simulink model "Copy_of_Mando"  (R2017b)
settings: Solver=FixedStepDiscrete  StartTime=0.0  StopTime=inf  FixedStep=0.001  MaxStep=1e-4  RelTol=1e-3  EnableMultiTasking=on
undefined symbols (not defined in the file): c_a, c_v, delta, Fc_mas_id, Fc_menos_id, Fs_mas_id, Fs_menos_id, Kp_c1, Kp_c2, Kp_h1, Kp_h2, Kv_c1, Kv_c2, Kv_h1, Kv_h2, nL, precision, sigma0_id, sigma1_id, sigma2_id, tau1, tfin, tini, vs_id
libraries: simulink x9, slrtlib x4, xpcnilib x3, dspbuff3 x2, vrlib x1, powerlib x1
settings Model: Creator=salas  LastModifiedBy=TrendingPC
settings OptimizationCC: LifeSpan=inf
settings DebuggingCC: SFUnexpectedBacktrackingDiag=warning  SFNoUnconditionalDefaultTransitionDiag=warning  SFExecutionAtInitializationDiag=none
settings CodeAppCC: StateflowObjectComments=on
settings GRTTargetCC: TargetLangStandard=C89/C90 (ANSI)  GeneratePreprocessorConditionals=Disable all
settings ConfigComp: CovMetricSettings=dw  CovHtmlReporting=on  CovSaveCumulativeToWorkspaceVar=on  CovSaveSingleToWorkspaceVar=on  CovExternalEMLEnable=off
settings SimscapeCC: SimscapeNormalizeSystem=off

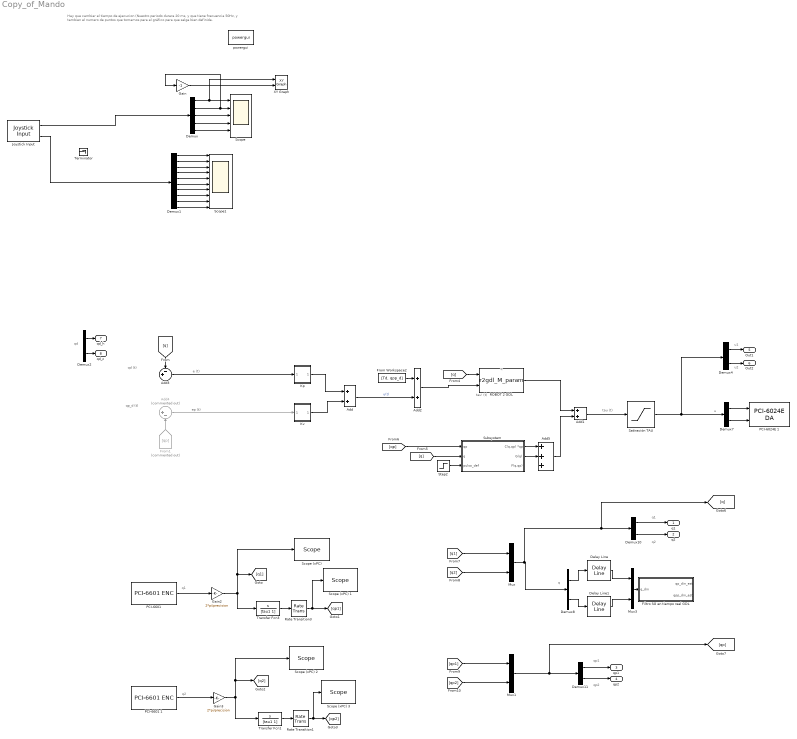
== system Copy_of_Mando ==
  note: Hay que cambiar el tiempo de ejecucion (Nuestro periodo durara 20 ms, y que tiene frecuencia 50Hz, y tambien el numero de puntos que tomamos para el gráfico para que salga bien definida.
  note: qd (t)
  note: q
  note: qd
  note: u1
  note: q2
  note: q2
  note: u2
  note: u
  note: qp2
  note: q1
  note: q
  note: qp_d (t)
  note: tau' (t)
  note: tau (t)
  note: e (t)
  note: q1
  note: ep (t)
  note: qp1
  Add : Sum
  Add1 : Sum
  Add2 : Sum
  Add3 : Sum  Inputs=-+|
  Add4 : Sum  Commented=on  Inputs=|+-
  Add5 : Sum  Inputs=+++
  Delay Line : dspbuff3/Delay Line  siz=nL+1  ic=0  directfeed=on  enable_output=off  hold_output=off  OutputFrames=on
      settings: SourceProductName=DSP System Toolbox  SourceProductBaseCode=DS
  Delay Line1 : dspbuff3/Delay Line  siz=nL+1  ic=0  directfeed=on  enable_output=off  hold_output=off  OutputFrames=on
      settings: SourceProductName=DSP System Toolbox  SourceProductBaseCode=DS
  Demux : Demux  Outputs=5
  Demux1 : Demux  Outputs=10
  Demux{2,4,7..8,10..11} (6 alike) : Demux  Outputs=2
  Filtro SG en tiempo real GDL : Subsystem
  From Workspace2 : FromWorkspace  VariableName=[Td, qpp_d]  SampleTime=0
  From1 : From  Commented=on  GotoTag=qp
      settings: CloseFcn=tagdialog Close
  Gain : Gain  Gain=-1
  Gain2 : Gain  Gain=2*pi/precision
  Gain3 : Gain  Gain=2*pi/precision
  Joystick Input : vrlib/Joystick Input  joyid=1  adjustports=on  forcefeed=off
      settings: SourceProductBaseCode=VR
  Kp : Subsystem
  Kv : Subsystem
  Mux : Mux  Inputs=2
  Mux1 : Mux  Inputs=2
  Mux3 : Mux  Inputs=2
  PCI-6024E 1 : xpcnilib/D//A/E Series/PCI-6024E DA  channel=[1,2]  reset=[1]  initValue=[0]  sampletime=0.001  slot=-1
      settings: SourceProductName=Simulink Real-Time  SourceProductBaseCode=XP
  "PCI-6601 " : xpcnilib/Incremental Encoder/PCI-6601 ENC  channel=1  countMode=Quadrature Mode X1  initCount=0  reload=off  indexPhase=A high B high  filter=None  sampleTime=0.001  slot=-1
      settings: SourceProductName=Simulink Real-Time  SourceProductBaseCode=XP
  PCI-6601 1 : xpcnilib/Incremental Encoder/PCI-6601 ENC  channel=2  countMode=Quadrature Mode X1  initCount=0  reload=off  indexPhase=A high B high  filter=None  sampleTime=0.001  slot=-1
      settings: SourceProductName=Simulink Real-Time  SourceProductBaseCode=XP
  ROBOT 2 GDL : S-Function  FunctionName=r2gdl_M_param  Parameters=k_id  SFunctionDeploymentMode=off  EnableBusSupport=off
  Rate Transition1 : RateTransition  OutPortSampleTime=0.001
  Rate Transition3 : RateTransition  OutPortSampleTime=0.001
  Satiración TAU : Saturate  UpperLimit=10  LowerLimit=-10  SampleTime=0.001
  Scope : Scope  NumInputPorts=5
  "Scope (xPC) " : slrtlib/Displays and Logging/Scope   scopeno=1  scopetype=Target  autostart=on  viewmode=Graphical redraw  formatstr='%15.6f'  grid=on  ylimits=[0,0]  nosamples=250  noprepostsamples=0  interleave=1  triggermode=FreeRun  triggersignal=1  trigsignalfromport=off  triggerlevel=0.0  triggerslope=Either  triggerscope=1  triggersample=0  filename=data.dat  mode=Lazy  writesize=512  autorestart=off  dynamicfilemode=off  maxwritefilesize=512*1024^2
  Scope (xPC) 1 : slrtlib/Displays and Logging/Scope   scopeno=2  scopetype=Target  autostart=on  viewmode=Graphical redraw  formatstr='%15.6f'  grid=on  ylimits=[0,0]  nosamples=250  noprepostsamples=0  interleave=1  triggermode=FreeRun  triggersignal=1  trigsignalfromport=off  triggerlevel=0.0  triggerslope=Either  triggerscope=1  triggersample=0  filename=data.dat  mode=Lazy  writesize=512  autorestart=off  dynamicfilemode=off  maxwritefilesize=512*1024^2
  Scope (xPC) 2 : slrtlib/Displays and Logging/Scope   scopeno=3  scopetype=Target  autostart=on  viewmode=Graphical redraw  formatstr='%15.6f'  grid=on  ylimits=[0,0]  nosamples=250  noprepostsamples=0  interleave=1  triggermode=FreeRun  triggersignal=1  trigsignalfromport=off  triggerlevel=0.0  triggerslope=Either  triggerscope=1  triggersample=0  filename=data.dat  mode=Lazy  writesize=512  autorestart=off  dynamicfilemode=off  maxwritefilesize=512*1024^2
  Scope (xPC) 3 : slrtlib/Displays and Logging/Scope   scopeno=4  scopetype=Target  autostart=on  viewmode=Graphical redraw  formatstr='%15.6f'  grid=on  ylimits=[0,0]  nosamples=250  noprepostsamples=0  interleave=1  triggermode=FreeRun  triggersignal=1  trigsignalfromport=off  triggerlevel=0.0  triggerslope=Either  triggerscope=1  triggersample=0  filename=data.dat  mode=Lazy  writesize=512  autorestart=off  dynamicfilemode=off  maxwritefilesize=512*1024^2
  Scope1 : Scope  NumInputPorts=10
  Step2 : Step  Time=0  SampleTime=0.001
  Subsystem : Subsystem
  Terminator : Terminator
  Transfer Fcn1 : TransferFcn  Numerator=[1 0]  Denominator=[tau1 1]
  Transfer Fcn3 : TransferFcn  Numerator=[1 0]  Denominator=[tau1 1]
  XY Graph : simulink/Sinks/XY Graph  xmin=-1  xmax=1  ymin=-1  ymax=1  st=-1
  powergui : powerlib/powergui  Priority=1  SimulationMode=Discrete  SampleTime=0.001  frequency=60  Iterations=50  frequencyindice=50  Pbase=100e6  ErrMax=1e-4  UnitsV=kV  UnitsW=MW  buscounter=0  FunctionMessages=off  echomessages=off  EnableUseOfTLC=off  CurrentSourceSwitches=off  DisableSnubberDevices=off  DisableRonSwitches=off  DisableVfSwitches=off  DisplayEquations=off  SolverType=Tustin/Backward Euler (TBE)  Interpol=off  ExternalGateDelay=off  methode=off  Ts=100  x0status=blocks  SPID=on  SwTol=0  HookPort=off  RestoreLinks=warning  ResistiveCurrentMeasurement=off  Frange=[0:2:500]  Ylog=off  Xlog=on  ShowGrid=off  save=off  variable=ZData  structure=0  ZoomFFT=off  StartTime=0.0  cycles=1  DisplayStyle=1  fundamental=60  FreqAxis=off  MaxFrequency=1000  frequencyindicesteady=1  RmsSteady=1  display=off
  q1 : Outport
  q2 : Outport  Port=2
  qp1 : Outport  Port=3
  qp2 : Outport  Port=4
  Out1 : Outport  Port=5
  Out2 : Outport  Port=6
  qd_h : Outport  Port=7
  qd_c : Outport  Port=8
  wires:
  Joystick Input/1 -> Demux/1
  Demux/1 -> XY Graph/1, Scope/1
  Demux/3 -> Scope/3
  Demux/4 -> Scope/4
  Demux/5 -> Scope/5
  Gain/1 -> XY Graph/2
  Demux/2 -> Gain/1, Scope/2
  Demux1/1 -> Scope1/1
  Demux1/2 -> Scope1/2
  Demux1/3 -> Scope1/3
  Demux1/4 -> Scope1/4
  Demux1/5 -> Scope1/5
  Demux1/6 -> Scope1/6
  Demux1/7 -> Scope1/7
  Demux1/8 -> Scope1/8
  Demux1/9 -> Scope1/9
  Demux1/10 -> Scope1/10
  Joystick Input/2 -> Demux1/1
  ? -> Terminator/1
  Demux10/1 -> q1/1
  Demux11/2 -> qp2/1
  Kv/1(Kp*e) -> Add/2
  "PCI-6601 "/1 -> Gain2/1
  Demux8/2 -> Delay Line1/1
  Demux7/1 -> PCI-6024E 1/1
  Rate Transition3/1 -> Scope (xPC) 1/1, [qp1]
  Mux1/1 -> [qp], Demux11/1
  Mux3/1 -> Filtro SG en tiempo real GDL/1(q_din)
  Add5/1 -> Add1/2
  Demux10/2 -> q2/1
  Transfer Fcn1/1 -> Rate Transition1/1
  [q] -> Add3/1
  [qp1] -> Mux1/1
  ? -> Demux2/1, Add3/2
  Gain2/1 -> Transfer Fcn3/1, "Scope (xPC) "/1, [q1]
  Demux2/1 -> qd_h/1
  [q] -> ROBOT 2 GDL/1
  Mux/1 -> Demux10/1, [q], Demux8/1
  Demux4/1 -> Out1/1
  Rate Transition1/1 -> Scope (xPC) 3/1, [qp2]
  Transfer Fcn3/1 -> Rate Transition3/1
  Delay Line/1 -> Mux3/1
  [qp2] -> Mux1/2
  Delay Line1/1 -> Mux3/2
  PCI-6601 1/1 -> Gain3/1
  [q2] -> Mux/2
  Demux8/1 -> Delay Line/1
  Demux2/2 -> qd_c/1
  Gain3/1 -> [q2], Scope (xPC) 2/1, Transfer Fcn1/1
  Subsystem/1(C(q,qp) *qp) -> Add5/1
  ROBOT 2 GDL/1 -> Add1/1
  Satiración TAU/1 -> Demux4/1, Demux7/1
  ? -> Add4/1
  Add2/1 -> ROBOT 2 GDL/2
  Demux7/2 -> PCI-6024E 1/2
  [qp] -> Subsystem/1(qp)
  Add3/1 -> Kp/1(e(t))
  Step2/1 -> Subsystem/3(pulso_def)
  Add/1 -> Add2/2  "u(t)"
  Demux4/2 -> Out2/1
  Add1/1 -> Satiración TAU/1
  Add4/1 -> Kv/1(e(t))
  Kp/1(Kp*e) -> Add/1
  [q1] -> Mux/1
  [q] -> Subsystem/2(q)
  Demux11/1 -> qp1/1
  From Workspace2/1 -> Add2/1
  Subsystem/2(G(q)) -> Add5/2
  From1/1 -> Add4/2

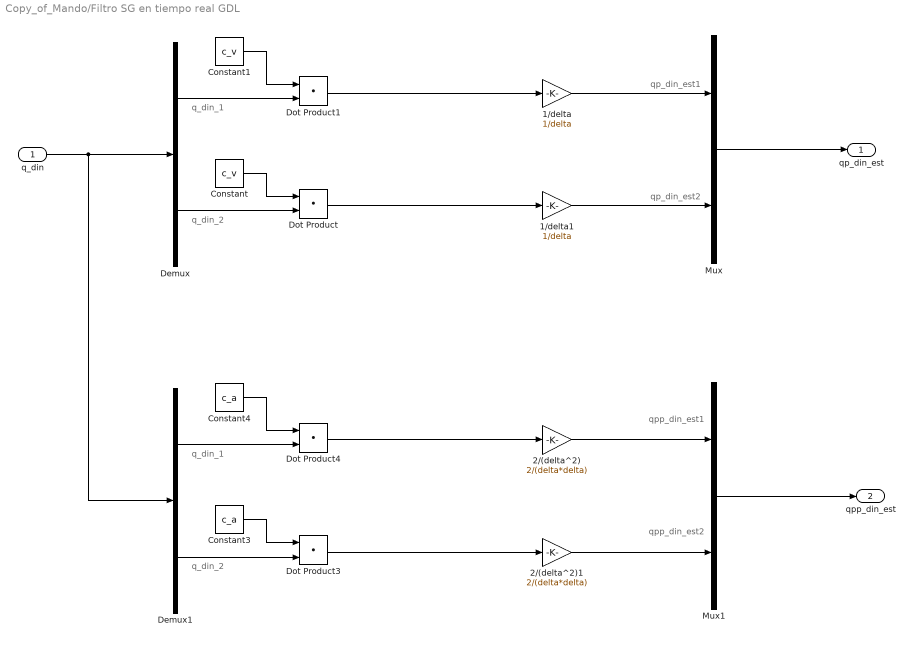
== system Copy_of_Mando/Filtro SG en tiempo real GDL ==
  note: q_din_2
  note: q_din_1
  note: qp_din_est1
  note: qp_din_est2
  note: q_din_2
  note: q_din_1
  note: qpp_din_est1
  note: qpp_din_est2
  q_din : Inport  SampleTime=0.001
  1/delta : Gain  Gain=1/delta  SampleTime=0.001
  1/delta1 : Gain  Gain=1/delta  SampleTime=0.001
  2/(delta^2) : Gain  Gain=2/(delta*delta)  SampleTime=0.001
  2/(delta^2)1 : Gain  Gain=2/(delta*delta)  SampleTime=0.001
  Constant : Constant  Value=c_v  SampleTime=0.001
  Constant1 : Constant  Value=c_v  SampleTime=0.001
  Constant3 : Constant  Value=c_a  VectorParams1D=off  SampleTime=0.001
  Constant4 : Constant  Value=c_a  SampleTime=0.001
  Demux : Demux  Outputs=2
  Demux1 : Demux  Outputs=2
  Dot Product{,1,3..4} (4 alike) : DotProduct  InputSameDT=on  OutDataTypeStr=Inherit: Inherit via internal rule
  Mux : Mux  Inputs=2
  Mux1 : Mux  Inputs=2
  qp_din_est : Outport  SampleTime=0.001
  qpp_din_est : Outport  Port=2  SampleTime=0.001
  wires:
  q_din/1 -> Demux/1, Demux1/1
  Constant1/1 -> Dot Product1/1
  Demux/1 -> Dot Product1/2
  1/delta/1 -> Mux/1
  1/delta1/1 -> Mux/2
  Mux/1 -> qp_din_est/1
  Dot Product/1 -> 1/delta1/1
  Dot Product1/1 -> 1/delta/1
  Demux/2 -> Dot Product/2
  Constant/1 -> Dot Product/1
  Constant4/1 -> Dot Product4/1
  Demux1/1 -> Dot Product4/2
  2/(delta^2)/1 -> Mux1/1
  2/(delta^2)1/1 -> Mux1/2
  Dot Product3/1 -> 2/(delta^2)1/1
  Dot Product4/1 -> 2/(delta^2)/1
  Demux1/2 -> Dot Product3/2
  Constant3/1 -> Dot Product3/1
  Mux1/1 -> qpp_din_est/1

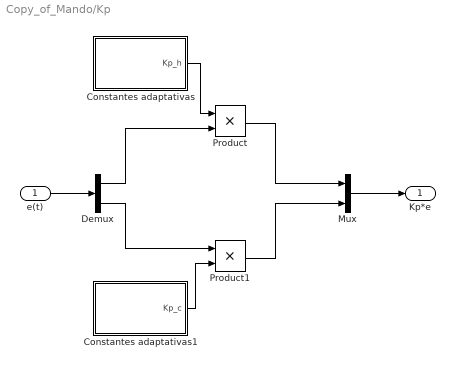
== system Copy_of_Mando/Kp ==
  e(t) : Inport
  Constantes adaptativas : Subsystem
  Constantes adaptativas1 : Subsystem
  Demux : Demux  Outputs=2
  Mux : Mux  Inputs=2
  Product : Product  RndMeth=Zero
  Product1 : Product  RndMeth=Zero
  Kp*e : Outport
  wires:
  Constantes adaptativas1/1(Kp_c) -> Product1/2
  Demux/2 -> Product1/1
  Product1/1 -> Mux/2
  Constantes adaptativas/1(Kp_h) -> Product/1
  Product/1 -> Mux/1
  Demux/1 -> Product/2
  Mux/1 -> Kp*e/1
  e(t)/1 -> Demux/1

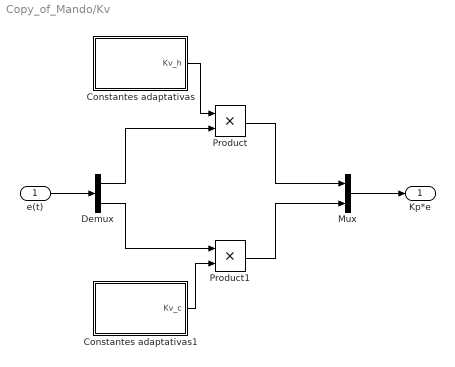
== system Copy_of_Mando/Kv ==
  e(t) : Inport
  Constantes adaptativas : Subsystem
  Constantes adaptativas1 : Subsystem
  Demux : Demux  Outputs=2
  Mux : Mux  Inputs=2
  Product : Product  RndMeth=Zero
  Product1 : Product  RndMeth=Zero
  Kp*e : Outport
  wires:
  e(t)/1 -> Demux/1
  Mux/1 -> Kp*e/1
  Demux/1 -> Product/2
  Product/1 -> Mux/1
  Constantes adaptativas/1(Kv_h) -> Product/1
  Product1/1 -> Mux/2
  Demux/2 -> Product1/1
  Constantes adaptativas1/1(Kv_c) -> Product1/2

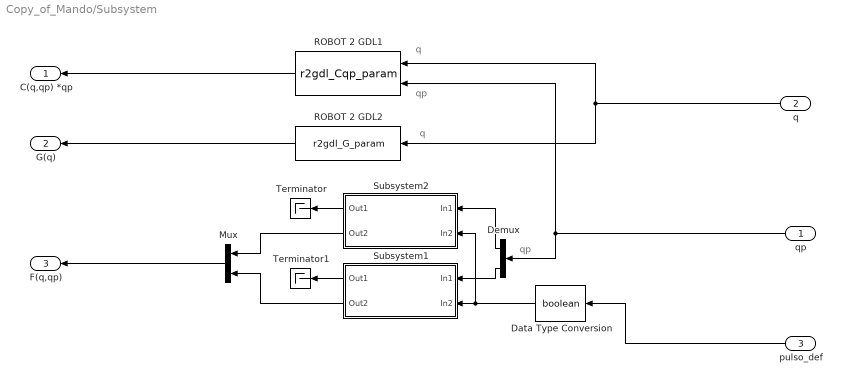
== system Copy_of_Mando/Subsystem ==
  note: qp
  note: q
  note: q
  note: qp
  qp : Inport
  q : Inport  Port=2
  pulso_def : Inport  Port=3
  Data Type Conversion : DataTypeConversion  OutDataTypeStr=boolean
  Demux : Demux  Outputs=2
  Mux : Mux  Inputs=2
  ROBOT 2 GDL1 : S-Function  FunctionName=r2gdl_Cqp_param  Parameters=k_id  SFunctionDeploymentMode=off  EnableBusSupport=off
  ROBOT 2 GDL2 : S-Function  FunctionName=r2gdl_G_param  Parameters=k_id  SFunctionDeploymentMode=off  EnableBusSupport=off
  Subsystem1 : Subsystem
      mask Display:
      | disp('Fricción Lugre')
      | port_label('output', 1, 'z')
      | port_label('output', 2, 'F')
      | port_label('input', 1, 'v')
  Subsystem2 : Subsystem
      mask Display:
      | disp('Fricción Lugre')
      | port_label('output', 1, 'z')
      | port_label('output', 2, 'F')
      | port_label('input', 1, 'v')
  Terminator : Terminator
  Terminator1 : Terminator
  C(q,qp) *qp : Outport
  G(q) : Outport  Port=2
  F(q,qp) : Outport  Port=3
  wires:
  Data Type Conversion/1 -> Subsystem2/2(In2), Subsystem1/2(In2)
  pulso_def/1 -> Data Type Conversion/1
  qp/1 -> ROBOT 2 GDL1/2, Demux/1
  q/1 -> ROBOT 2 GDL2/1, ROBOT 2 GDL1/1
  Mux/1 -> F(q,qp)/1
  ROBOT 2 GDL2/1 -> G(q)/1
  ROBOT 2 GDL1/1 -> C(q,qp) *qp/1
  Subsystem1/1(Out1) -> Terminator1/1
  Subsystem1/2(Out2) -> Mux/2
  Subsystem2/2(Out2) -> Mux/1
  Demux/2 -> Subsystem1/1(In1)
  Demux/1 -> Subsystem2/1(In1)
  Subsystem2/1(Out1) -> Terminator/1

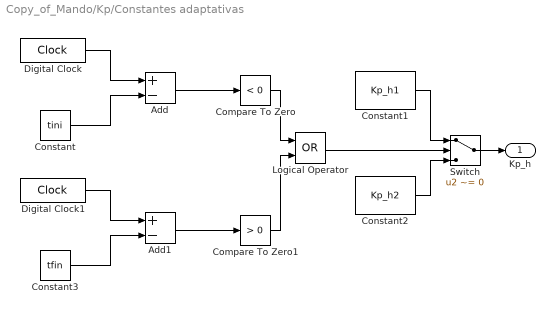
== system Copy_of_Mando/Kp/Constantes adaptativas ==
  Add : Sum  Inputs=+-
  Add1 : Sum  Inputs=+-
  Compare To Zero : simulink/Logic and Bit Operations/Compare To Zero  relop=<  OutDataTypeStr=uint8  ZeroCross=off
  Compare To Zero1 : simulink/Logic and Bit Operations/Compare To Zero  relop=>  OutDataTypeStr=uint8  ZeroCross=off
  Constant : Constant  Value=tini
  Constant1 : Constant  Value=Kp_h1
  Constant2 : Constant  Value=Kp_h2
  Constant3 : Constant  Value=tfin
  Digital Clock : DigitalClock  SampleTime=0.001
  Digital Clock1 : DigitalClock  SampleTime=0.001
  Logical Operator : Logic  Operator=OR  AllPortsSameDT=off  OutDataTypeStr=boolean
  Switch : Switch  Criteria=u2 ~= 0
  Kp_h : Outport
  wires:
  Switch/1 -> Kp_h/1
  Compare To Zero1/1 -> Logical Operator/2
  Compare To Zero/1 -> Logical Operator/1
  Logical Operator/1 -> Switch/2
  Add1/1 -> Compare To Zero1/1
  Constant3/1 -> Add1/2
  Digital Clock1/1 -> Add1/1
  Constant1/1 -> Switch/1
  Constant2/1 -> Switch/3
  Add/1 -> Compare To Zero/1
  Constant/1 -> Add/2
  Digital Clock/1 -> Add/1

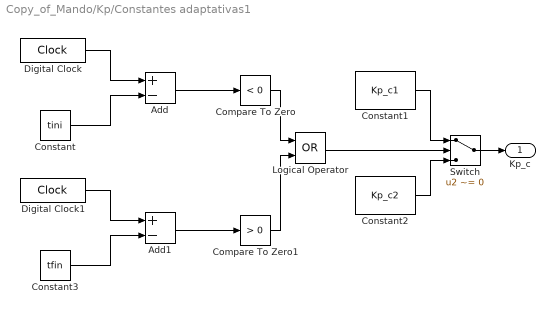
== system Copy_of_Mando/Kp/Constantes adaptativas1 ==
  Add : Sum  Inputs=+-
  Add1 : Sum  Inputs=+-
  Compare To Zero : simulink/Logic and Bit Operations/Compare To Zero  relop=<  OutDataTypeStr=uint8  ZeroCross=off
  Compare To Zero1 : simulink/Logic and Bit Operations/Compare To Zero  relop=>  OutDataTypeStr=uint8  ZeroCross=off
  Constant : Constant  Value=tini
  Constant1 : Constant  Value=Kp_c1
  Constant2 : Constant  Value=Kp_c2
  Constant3 : Constant  Value=tfin
  Digital Clock : DigitalClock  SampleTime=0.001
  Digital Clock1 : DigitalClock  SampleTime=0.001
  Logical Operator : Logic  Operator=OR  AllPortsSameDT=off  OutDataTypeStr=boolean
  Switch : Switch  Criteria=u2 ~= 0
  Kp_c : Outport
  wires:
  Digital Clock/1 -> Add/1
  Constant/1 -> Add/2
  Add/1 -> Compare To Zero/1
  Constant2/1 -> Switch/3
  Constant1/1 -> Switch/1
  Digital Clock1/1 -> Add1/1
  Constant3/1 -> Add1/2
  Add1/1 -> Compare To Zero1/1
  Logical Operator/1 -> Switch/2
  Compare To Zero/1 -> Logical Operator/1
  Compare To Zero1/1 -> Logical Operator/2
  Switch/1 -> Kp_c/1

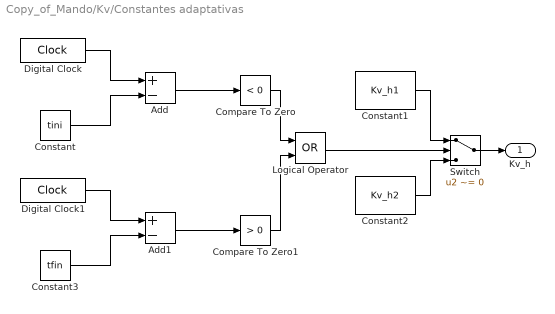
== system Copy_of_Mando/Kv/Constantes adaptativas ==
  Add : Sum  Inputs=+-
  Add1 : Sum  Inputs=+-
  Compare To Zero : simulink/Logic and Bit Operations/Compare To Zero  relop=<  OutDataTypeStr=uint8  ZeroCross=off
  Compare To Zero1 : simulink/Logic and Bit Operations/Compare To Zero  relop=>  OutDataTypeStr=uint8  ZeroCross=off
  Constant : Constant  Value=tini
  Constant1 : Constant  Value=Kv_h1
  Constant2 : Constant  Value=Kv_h2
  Constant3 : Constant  Value=tfin
  Digital Clock : DigitalClock  SampleTime=0.001
  Digital Clock1 : DigitalClock  SampleTime=0.001
  Logical Operator : Logic  Operator=OR  AllPortsSameDT=off  OutDataTypeStr=boolean
  Switch : Switch  Criteria=u2 ~= 0
  Kv_h : Outport
  wires:
  Digital Clock/1 -> Add/1
  Constant/1 -> Add/2
  Add/1 -> Compare To Zero/1
  Constant2/1 -> Switch/3
  Constant1/1 -> Switch/1
  Digital Clock1/1 -> Add1/1
  Constant3/1 -> Add1/2
  Add1/1 -> Compare To Zero1/1
  Logical Operator/1 -> Switch/2
  Compare To Zero/1 -> Logical Operator/1
  Compare To Zero1/1 -> Logical Operator/2
  Switch/1 -> Kv_h/1

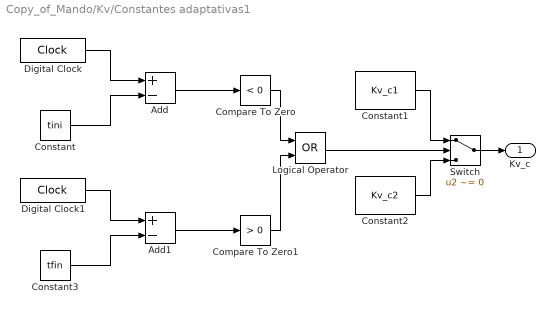
== system Copy_of_Mando/Kv/Constantes adaptativas1 ==
  Add : Sum  Inputs=+-
  Add1 : Sum  Inputs=+-
  Compare To Zero : simulink/Logic and Bit Operations/Compare To Zero  relop=<  OutDataTypeStr=uint8  ZeroCross=off
  Compare To Zero1 : simulink/Logic and Bit Operations/Compare To Zero  relop=>  OutDataTypeStr=uint8  ZeroCross=off
  Constant : Constant  Value=tini
  Constant1 : Constant  Value=Kv_c1
  Constant2 : Constant  Value=Kv_c2
  Constant3 : Constant  Value=tfin
  Digital Clock : DigitalClock  SampleTime=0.001
  Digital Clock1 : DigitalClock  SampleTime=0.001
  Logical Operator : Logic  Operator=OR  AllPortsSameDT=off  OutDataTypeStr=boolean
  Switch : Switch  Criteria=u2 ~= 0
  Kv_c : Outport
  wires:
  Switch/1 -> Kv_c/1
  Compare To Zero1/1 -> Logical Operator/2
  Compare To Zero/1 -> Logical Operator/1
  Logical Operator/1 -> Switch/2
  Add1/1 -> Compare To Zero1/1
  Constant3/1 -> Add1/2
  Digital Clock1/1 -> Add1/1
  Constant1/1 -> Switch/1
  Constant2/1 -> Switch/3
  Add/1 -> Compare To Zero/1
  Constant/1 -> Add/2
  Digital Clock/1 -> Add/1

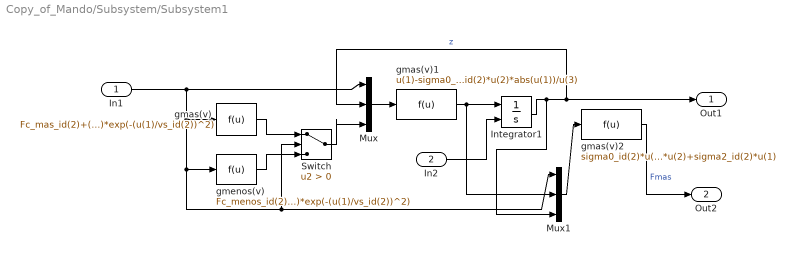
== system Copy_of_Mando/Subsystem/Subsystem1 ==
  In1 : Inport
  In2 : Inport  Port=2
  Integrator1 : Integrator  ExternalReset=rising
  Mux : Mux  Inputs=3
  Mux1 : Mux  Inputs=3
  Switch : Switch  Criteria=u2 > Threshold
  gmas(v) : Fcn  Expr=Fc_mas_id(2)+(Fs_mas_id(2)-Fc_mas_id(2))*exp(-(u(1)/vs_id(2))^2)
  gmas(v)1 : Fcn  Expr=u(1)-sigma0_id(2)*u(2)*abs(u(1))/u(3)
  gmas(v)2 : Fcn  Expr=sigma0_id(2)*u(3)+sigma1_id(2)*u(2)+sigma2_id(2)*u(1)
  gmenos(v) : Fcn  Expr=Fc_menos_id(2)+(Fs_menos_id(2)-Fc_menos_id(2))*exp(-(u(1)/vs_id(2))^2)
  Out1 : Outport
  Out2 : Outport  Port=2
  wires:
  In2/1 -> Integrator1/2
  gmas(v)1/1 -> Integrator1/1, Mux1/2
  Integrator1/1 -> Mux/2, Out1/1, Mux1/3  "z"
  In1/1 -> Mux/1, gmas(v)/1, gmenos(v)/1, Mux1/1, Switch/2
  Mux/1 -> gmas(v)1/1
  Mux1/1 -> gmas(v)2/1
  Switch/1 -> Mux/3
  gmas(v)/1 -> Switch/1
  gmenos(v)/1 -> Switch/3
  gmas(v)2/1 -> Out2/1  "Fmas"

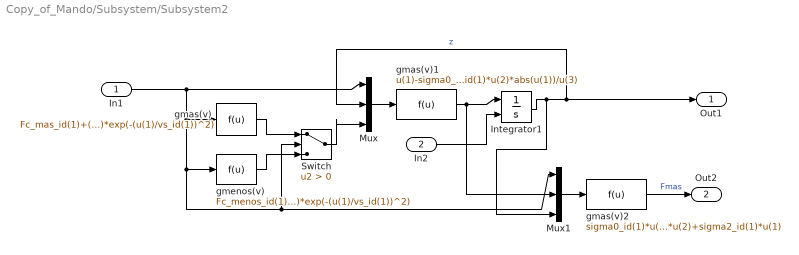
== system Copy_of_Mando/Subsystem/Subsystem2 ==
  In1 : Inport
  In2 : Inport  Port=2
  Integrator1 : Integrator  ExternalReset=rising
  Mux : Mux  Inputs=3
  Mux1 : Mux  Inputs=3
  Switch : Switch  Criteria=u2 > Threshold
  gmas(v) : Fcn  Expr=Fc_mas_id(1)+(Fs_mas_id(1)-Fc_mas_id(1))*exp(-(u(1)/vs_id(1))^2)
  gmas(v)1 : Fcn  Expr=u(1)-sigma0_id(1)*u(2)*abs(u(1))/u(3)
  gmas(v)2 : Fcn  Expr=sigma0_id(1)*u(3)+sigma1_id(1)*u(2)+sigma2_id(1)*u(1)
  gmenos(v) : Fcn  Expr=Fc_menos_id(1)+(Fs_menos_id(1)-Fc_menos_id(1))*exp(-(u(1)/vs_id(1))^2)
  Out1 : Outport
  Out2 : Outport  Port=2
  wires:
  In2/1 -> Integrator1/2
  gmas(v)2/1 -> Out2/1  "Fmas"
  gmenos(v)/1 -> Switch/3
  gmas(v)/1 -> Switch/1
  Switch/1 -> Mux/3
  Mux1/1 -> gmas(v)2/1
  Mux/1 -> gmas(v)1/1
  In1/1 -> Switch/2, Mux1/1, gmenos(v)/1, gmas(v)/1, Mux/1
  Integrator1/1 -> Mux1/3, Out1/1, Mux/2  "z"
  gmas(v)1/1 -> Mux1/2, Integrator1/1
